simulink model "smartCart5_1work"  (R2016a)
settings: Solver=FixedStepDiscrete  StartTime=0.0  StopTime=inf  FixedStep=1  RelTol=1e-3
libraries: simulink x213, hdlsllib x84
(part 4 of 4)

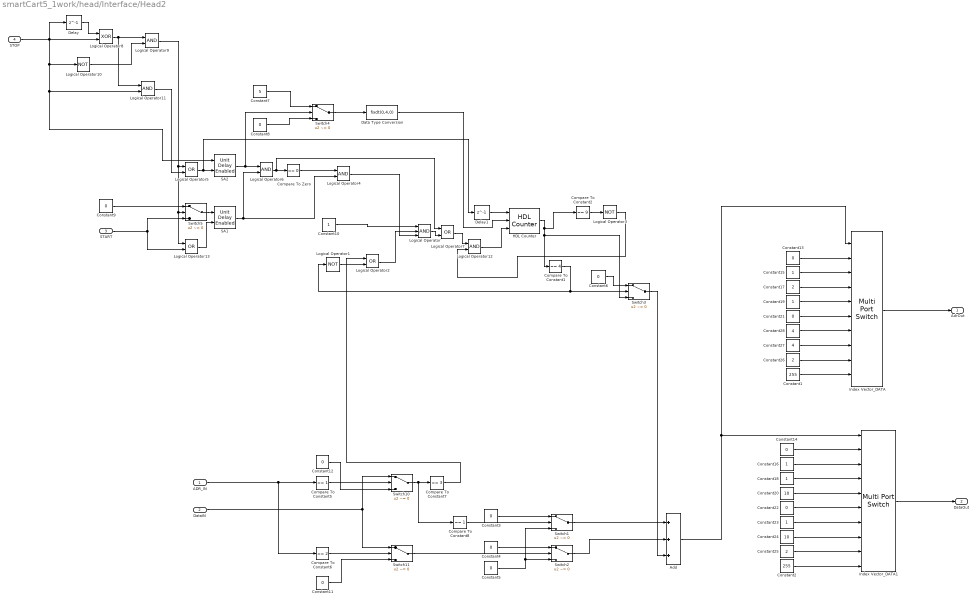
== system smartCart5_1work/head/Interface/Head2 ==
  ADR_IN : Inport  OutDataTypeStr=uint8
  DataIN : Inport  Port=2  OutDataTypeStr=uint8
  START : Inport  Port=3  OutDataTypeStr=boolean
  STOP : Inport  Port=4  OutDataTypeStr=boolean
  Add : Sum  Inputs=+++
  Compare To Constant1 : simulink/Logic and Bit Operations/Compare To Constant  relop===  const=4  OutDataTypeStr=boolean
  Compare To Constant2 : simulink/Logic and Bit Operations/Compare To Constant  relop===  const=9  OutDataTypeStr=boolean
  Compare To Constant5 : simulink/Logic and Bit Operations/Compare To Constant  relop===  const=1  OutDataTypeStr=boolean
  Compare To Constant6 : simulink/Logic and Bit Operations/Compare To Constant  relop===  const=2  OutDataTypeStr=boolean
  Compare To Constant7 : simulink/Logic and Bit Operations/Compare To Constant  relop===  const=3  OutDataTypeStr=boolean
  Compare To Constant8 : simulink/Logic and Bit Operations/Compare To Constant  relop===  const=1  OutDataTypeStr=boolean
  Compare To Zero : simulink/Logic and Bit Operations/Compare To Zero  relop===  OutDataTypeStr=boolean
  Constant1 : Constant  Value=255  OutDataTypeStr=uint8
  Constant10 : Constant  OutDataTypeStr=boolean
  Constant{3..6,11..14,21..22} (10 alike) : Constant  Value=0  OutDataTypeStr=uint8
  Constant{15..16,18..19,23} (5 alike) : Constant  OutDataTypeStr=uint8
  Constant17 : Constant  Value=2  OutDataTypeStr=uint8
  Constant2 : Constant  Value=255  OutDataTypeStr=uint8
  Constant20 : Constant  Value=10  OutDataTypeStr=uint8
  Constant24 : Constant  Value=10  OutDataTypeStr=uint8
  Constant25 : Constant  Value=2  OutDataTypeStr=uint8
  Constant26 : Constant  Value=2  OutDataTypeStr=uint8
  Constant27 : Constant  Value=4  OutDataTypeStr=uint8
  Constant28 : Constant  Value=4  OutDataTypeStr=uint8
  Constant7 : Constant  Value=5  OutDataTypeStr=fixdt(0,4,0)
  Constant8 : Constant  Value=0  OutDataTypeStr=fixdt(0,4,0)
  Constant9 : Constant  Value=0  OutDataTypeStr=boolean
  Data Type Conversion : DataTypeConversion  OutDataTypeStr=fixdt(0,4,0)
  Delay : Delay  DelayLength=1  InitialCondition=0
  Delay1 : Delay  DelayLength=1  InitialCondition=0
  HDL Counter : hdlsllib/HDL Operations/HDL Counter  CountType=Free running  CountInit=0  CountStep=1  CountMax=100  CountFromType=Initial value  CountFrom=0  CountResetPort=off  CountLoadPort=on  CountEnbPort=on  CountDirPort=off  CountDataType=Unsigned  CountWordLen=4  CountFracLen=0  CountSampTime=1
  Index Vector_DATA : MultiPortSwitch  DataPortOrder=Zero-based contiguous  Inputs=9  DiagnosticForDefault=None  zeroidx=on  OutDataTypeStr=uint8
  Index Vector_DATA1 : MultiPortSwitch  DataPortOrder=Zero-based contiguous  Inputs=9  DiagnosticForDefault=None  zeroidx=on  OutDataTypeStr=uint8
  Logical Operator : Logic  Inputs=3  AllPortsSameDT=off  OutDataTypeStr=boolean
  Logical Operator1 : Logic  Operator=NOT  AllPortsSameDT=off  OutDataTypeStr=boolean
  Logical Operator10 : Logic  Operator=NOT  AllPortsSameDT=off  OutDataTypeStr=boolean
  Logical Operator{4,6,9,11..12} (5 alike) : Logic  AllPortsSameDT=off  OutDataTypeStr=boolean
  Logical Operator{2,5,7,13} (4 alike) : Logic  Operator=OR  AllPortsSameDT=off  OutDataTypeStr=boolean
  Logical Operator3 : Logic  Operator=NOT  AllPortsSameDT=off  OutDataTypeStr=boolean
  Logical Operator8 : Logic  Operator=XOR  AllPortsSameDT=off  OutDataTypeStr=boolean
  SA1 : simulink/Additional Math & Discrete/Additional Discrete/Unit Delay Enabled  vinit=0  tsamp=-1
  SA2 : simulink/Additional Math & Discrete/Additional Discrete/Unit Delay Enabled  vinit=0  tsamp=-1
  Switch{1..5,10..11} (7 alike) : Switch  Criteria=u2 ~= 0  OutDataTypeStr=uint8
  AdrOut : Outport  OutDataTypeStr=uint8
  DataOut : Outport  Port=2  OutDataTypeStr=uint8
  wires:
  Constant10/1 -> Logical Operator/1
  Compare To Constant5/1 -> Switch10/2
  Compare To Constant6/1 -> Switch11/2
  Constant11/1 -> Switch11/3
  Constant12/1 -> Switch10/3
  Switch10/1 -> Compare To Constant8/1, Compare To Constant7/1
  Constant13/1 -> Index Vector_DATA/2
  Constant14/1 -> Index Vector_DATA1/2
  Constant15/1 -> Index Vector_DATA/3
  Constant16/1 -> Index Vector_DATA1/3
  Constant17/1 -> Index Vector_DATA/4
  Constant18/1 -> Index Vector_DATA1/4
  Constant19/1 -> Index Vector_DATA/5
  Constant20/1 -> Index Vector_DATA1/5
  Constant21/1 -> Index Vector_DATA/6
  Constant22/1 -> Index Vector_DATA1/6
  Constant23/1 -> Index Vector_DATA1/7
  Constant24/1 -> Index Vector_DATA1/8
  Constant25/1 -> Index Vector_DATA1/9
  Constant26/1 -> Index Vector_DATA/9
  Constant27/1 -> Index Vector_DATA/8
  Constant28/1 -> Index Vector_DATA/7
  Compare To Constant1/1 -> Logical Operator1/1, Switch3/2
  Compare To Constant7/1 -> Logical Operator2/1
  Logical Operator1/1 -> Logical Operator2/2
  Constant1/1 -> Index Vector_DATA/10
  Constant2/1 -> Index Vector_DATA1/10
  Logical Operator2/1 -> Logical Operator/2
  Compare To Constant8/1 -> Switch1/2
  Constant3/1 -> Switch1/1
  Switch11/1 -> Switch2/2
  Constant4/1 -> Switch2/1
  HDL Counter/1 -> Compare To Constant2/1, Switch3/3, Compare To Constant1/1
  Constant5/1 -> Switch1/3, Switch2/3
  Constant6/1 -> Switch3/1
  Switch1/1 -> Add/1
  Switch2/1 -> Add/2
  Switch3/1 -> Add/3
  Add/1 -> Index Vector_DATA/1, Index Vector_DATA1/1
  Index Vector_DATA1/1 -> DataOut/1
  Index Vector_DATA/1 -> AdrOut/1
  ADR_IN/1 -> Compare To Constant5/1, Compare To Constant6/1
  DataIN/1 -> Switch11/1, Switch10/1
  Compare To Constant2/1 -> Logical Operator3/1
  Compare To Zero/1 -> Logical Operator4/1
  SA1/1 -> Logical Operator6/2, Logical Operator4/2
  Logical Operator4/1 -> Logical Operator/3
  Logical Operator/1 -> Logical Operator7/2
  STOP/1 -> SA2/1, Logical Operator11/2, Logical Operator10/1, Delay/1, Logical Operator8/2
  Delay/1 -> Logical Operator8/1
  Logical Operator8/1 -> Logical Operator11/1, Logical Operator9/1
  Logical Operator10/1 -> Logical Operator9/2
  Logical Operator5/1 -> Delay1/1, SA2/2
  Logical Operator11/1 -> Logical Operator5/2
  Logical Operator9/1 -> Logical Operator13/1, Switch5/2, Logical Operator5/1
  SA2/1 -> Switch4/2, Logical Operator6/1
  Logical Operator6/1 -> Logical Operator7/1, Compare To Zero/1
  Constant7/1 -> Switch4/1
  Constant8/1 -> Switch4/3
  Switch4/1 -> Data Type Conversion/1
  Data Type Conversion/1 -> HDL Counter/2
  Delay1/1 -> HDL Counter/1
  Logical Operator12/1 -> HDL Counter/3
  Logical Operator3/1 -> Logical Operator12/2
  Logical Operator7/1 -> Logical Operator12/1
  Switch5/1 -> SA1/1
  Constant9/1 -> Switch5/1
  START/1 -> Logical Operator13/2, Switch5/3
  Logical Operator13/1 -> SA1/2

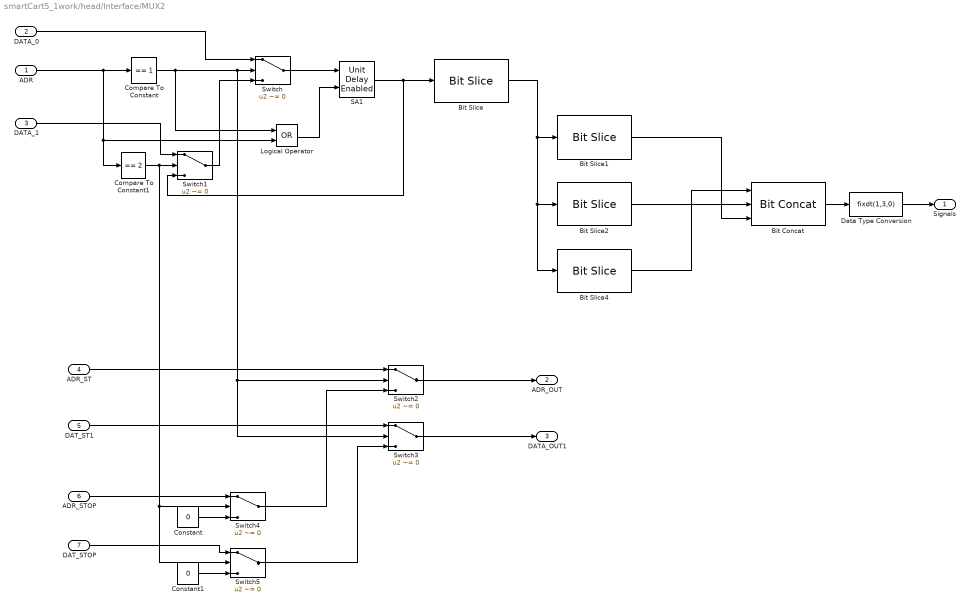
== system smartCart5_1work/head/Interface/MUX2 ==
  ADR : Inport  OutDataTypeStr=uint8
  DATA_0 : Inport  Port=2  OutDataTypeStr=uint8
  DATA_1 : Inport  Port=3  OutDataTypeStr=uint8
  ADR_ST : Inport  Port=4  OutDataTypeStr=uint8
  DAT_ST1 : Inport  Port=5  OutDataTypeStr=uint8
  ADR_STOP : Inport  Port=6  OutDataTypeStr=uint8
  DAT_STOP : Inport  Port=7  OutDataTypeStr=uint8
  Bit Concat : hdlsllib/HDL Operations/Bit Concat  numInputs=3
  Bit Slice : hdlsllib/HDL Operations/Bit Slice  lidx=4  ridx=0
  Bit Slice1 : hdlsllib/HDL Operations/Bit Slice  lidx=0  ridx=0
  Bit Slice2 : hdlsllib/HDL Operations/Bit Slice  lidx=1  ridx=1
  Bit Slice4 : hdlsllib/HDL Operations/Bit Slice  lidx=3  ridx=3
  Compare To Constant : simulink/Logic and Bit Operations/Compare To Constant  relop===  const=1  OutDataTypeStr=boolean
  Compare To Constant1 : simulink/Logic and Bit Operations/Compare To Constant  relop===  const=2  OutDataTypeStr=boolean
  Constant : Constant  Value=0  OutDataTypeStr=boolean
  Constant1 : Constant  Value=0  OutDataTypeStr=boolean
  Data Type Conversion : DataTypeConversion  OutDataTypeStr=fixdt(1,3,0)
  Logical Operator : Logic  Operator=OR  AllPortsSameDT=off  OutDataTypeStr=boolean
  SA1 : simulink/Additional Math & Discrete/Additional Discrete/Unit Delay Enabled  vinit=0  tsamp=-1
  Switch{,1..5} (6 alike) : Switch  Criteria=u2 ~= 0  OutDataTypeStr=uint8
  Signals : Outport  OutDataTypeStr=fixdt(1,3,0)
  ADR_OUT : Outport  Port=2  OutDataTypeStr=uint8
  DATA_OUT1 : Outport  Port=3  OutDataTypeStr=uint8
  wires:
  Bit Slice/1 -> Bit Slice4/1, Bit Slice2/1, Bit Slice1/1
  Compare To Constant/1 -> Logical Operator/1, Switch2/2, Switch3/2, Switch/2
  Switch1/1 -> Switch/3
  Compare To Constant1/1 -> Switch1/2, Switch4/2, Switch5/2
  Switch/1 -> SA1/1
  SA1/1 -> Bit Slice/1, Switch1/3
  Switch4/1 -> Switch2/3
  Switch5/1 -> Switch3/3
  Constant/1 -> Switch4/3
  Constant1/1 -> Switch5/3
  Logical Operator/1 -> SA1/2
  Switch2/1 -> ADR_OUT/1
  Switch3/1 -> DATA_OUT1/1
  DATA_0/1 -> Switch/1
  ADR/1 -> Logical Operator/2, Compare To Constant1/1, Compare To Constant/1
  DATA_1/1 -> Switch1/1
  ADR_ST/1 -> Switch2/1
  DAT_ST1/1 -> Switch3/1
  ADR_STOP/1 -> Switch4/1
  DAT_STOP/1 -> Switch5/1
  Bit Slice4/1 -> Bit Concat/1
  Bit Slice2/1 -> Bit Concat/2
  Bit Slice1/1 -> Bit Concat/3
  Bit Concat/1 -> Data Type Conversion/1
  Data Type Conversion/1 -> Signals/1

== system smartCart5_1work/head/Interface/Swith_signal2 ==
  Adr : Inport  OutDataTypeStr=uint8
  Data : Inport  Port=2  OutDataTypeStr=uint8
  Compare To Constant : simulink/Logic and Bit Operations/Compare To Constant  relop===  const=2  OutDataTypeStr=boolean
  SA1 : simulink/Additional Math & Discrete/Additional Discrete/Unit Delay Enabled  vinit=0  tsamp=-1
  OutAddr : Outport  OutDataTypeStr=uint8
  wires:
  Compare To Constant/1 -> SA1/2
  Adr/1 -> Compare To Constant/1
  Data/1 -> SA1/1
  SA1/1 -> OutAddr/1

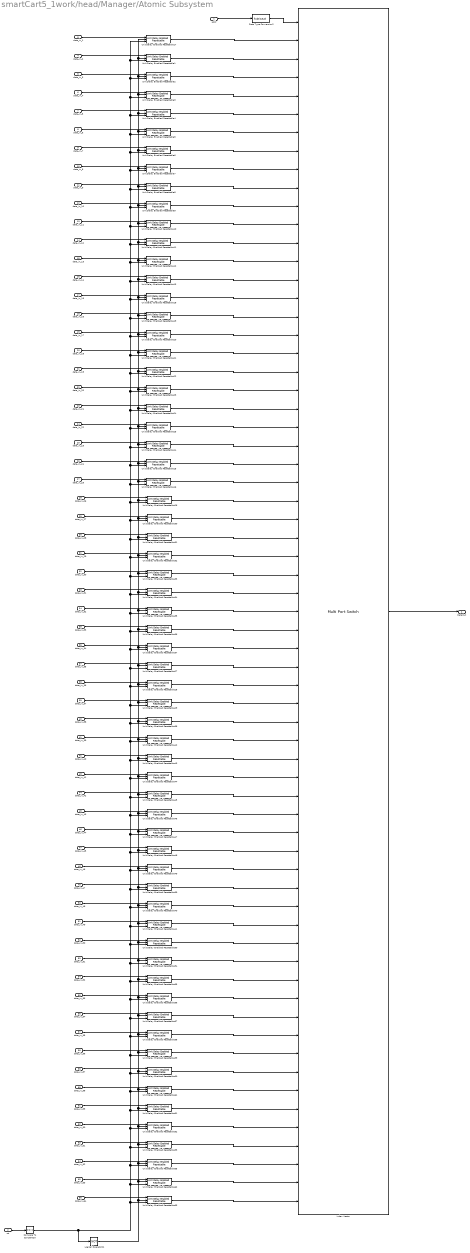
== system smartCart5_1work/head/Manager/Atomic Subsystem ==
  addr : Inport  OutDataTypeStr=uint8
  rst : Inport  Port=2  OutDataTypeStr=boolean
  data_in_1 : Inport  Port=3  OutDataTypeStr=uint32
  data_in_2 : Inport  Port=4  OutDataTypeStr=uint32
  data_in_3 : Inport  Port=5  OutDataTypeStr=uint32
  data_in_4 : Inport  Port=6  OutDataTypeStr=uint32
  data_in_5 : Inport  Port=7  OutDataTypeStr=uint32
  data_in_6 : Inport  Port=8  OutDataTypeStr=uint32
  data_in_7 : Inport  Port=9  OutDataTypeStr=uint32
  data_in_8 : Inport  Port=10  OutDataTypeStr=uint32
  data_in_9 : Inport  Port=11  OutDataTypeStr=uint32
  data_in_10 : Inport  Port=12  OutDataTypeStr=uint32
  data_in_11 : Inport  Port=13  OutDataTypeStr=uint32
  data_in_12 : Inport  Port=14  OutDataTypeStr=uint32
  data_in_13 : Inport  Port=15  OutDataTypeStr=uint32
  data_in_14 : Inport  Port=16  OutDataTypeStr=uint32
  data_in_15 : Inport  Port=17  OutDataTypeStr=uint32
  data_in_16 : Inport  Port=18  OutDataTypeStr=uint32
  data_in_17 : Inport  Port=19  OutDataTypeStr=uint32
  data_in_18 : Inport  Port=20  OutDataTypeStr=uint32
  data_in_19 : Inport  Port=21  OutDataTypeStr=uint32
  data_in_20 : Inport  Port=22  OutDataTypeStr=uint32
  data_in_21 : Inport  Port=23  OutDataTypeStr=uint32
  data_in_22 : Inport  Port=24  OutDataTypeStr=uint32
  data_in_23 : Inport  Port=25  OutDataTypeStr=uint32
  data_in_24 : Inport  Port=26  OutDataTypeStr=uint32
  data_in_25 : Inport  Port=27  OutDataTypeStr=uint32
  data_in_26 : Inport  Port=28  OutDataTypeStr=uint32
  data_in_27 : Inport  Port=29  OutDataTypeStr=uint32
  data_in_28 : Inport  Port=30  OutDataTypeStr=uint32
  data_in_29 : Inport  Port=31  OutDataTypeStr=uint32
  data_in_30 : Inport  Port=32  OutDataTypeStr=uint32
  data_in_31 : Inport  Port=33  OutDataTypeStr=uint32
  data_in_32 : Inport  Port=34  OutDataTypeStr=uint32
  data_in_33 : Inport  Port=35  OutDataTypeStr=uint32
  data_in_34 : Inport  Port=36  OutDataTypeStr=uint32
  data_in_35 : Inport  Port=37  OutDataTypeStr=uint32
  data_in_36 : Inport  Port=38  OutDataTypeStr=uint32
  data_in_37 : Inport  Port=39  OutDataTypeStr=uint32
  data_in_38 : Inport  Port=40  OutDataTypeStr=uint32
  data_in_39 : Inport  Port=41  OutDataTypeStr=uint32
  data_in_40 : Inport  Port=42  OutDataTypeStr=uint32
  data_in_41 : Inport  Port=43  OutDataTypeStr=uint32
  data_in_42 : Inport  Port=44  OutDataTypeStr=uint32
  data_in_43 : Inport  Port=45  OutDataTypeStr=uint32
  data_in_44 : Inport  Port=46  OutDataTypeStr=uint32
  data_in_45 : Inport  Port=47  OutDataTypeStr=uint32
  data_in_46 : Inport  Port=48  OutDataTypeStr=uint32
  data_in_47 : Inport  Port=49  OutDataTypeStr=uint32
  data_in_48 : Inport  Port=50  OutDataTypeStr=uint32
  data_in_49 : Inport  Port=51  OutDataTypeStr=uint32
  data_in_50 : Inport  Port=52  OutDataTypeStr=uint32
  data_in_51 : Inport  Port=53  OutDataTypeStr=uint32
  data_in_52 : Inport  Port=54  OutDataTypeStr=uint32
  data_in_53 : Inport  Port=55  OutDataTypeStr=uint32
  data_in_54 : Inport  Port=56  OutDataTypeStr=uint32
  data_in_55 : Inport  Port=57  OutDataTypeStr=uint32
  data_in_56 : Inport  Port=58  OutDataTypeStr=uint32
  data_in_57 : Inport  Port=59  OutDataTypeStr=uint32
  data_in_58 : Inport  Port=60  OutDataTypeStr=uint32
  data_in_59 : Inport  Port=61  OutDataTypeStr=uint32
  data_in_60 : Inport  Port=62  OutDataTypeStr=uint32
  data_in_61 : Inport  Port=63  OutDataTypeStr=uint32
  data_in_62 : Inport  Port=64  OutDataTypeStr=uint32
  data_in_63 : Inport  Port=65  OutDataTypeStr=uint32
  data_in_64 : Inport  Port=66  OutDataTypeStr=uint32
  Compare To Constant20 : simulink/Logic and Bit Operations/Compare To Constant  relop===  const=1  OutDataTypeStr=boolean
  Data Type Conversion2 : DataTypeConversion  OutDataTypeStr=fixdt(0,6,0)
  Index Vector : MultiPortSwitch  DataPortOrder=Zero-based contiguous  Inputs=64  zeroidx=on
  Logical Operator21 : Logic  Operator=NOT  AllPortsSameDT=off  OutDataTypeStr=boolean
  Unit Delay Enabled Resettable{1..63,65} (64 alike) : simulink/Additional Math & Discrete/Additional Discrete/Unit Delay Enabled Resettable  vinit=0  tsamp=-1
  DataOut : Outport  OutDataTypeStr=uint32
  wires:
  addr/1 -> Data Type Conversion2/1
  data_in_1/1 -> Unit Delay Enabled Resettable17/1
  Unit Delay Enabled Resettable17/1 -> Index Vector/2
  rst/1 -> Compare To Constant20/1
  Unit Delay Enabled Resettable1/1 -> Index Vector/3
  Unit Delay Enabled Resettable2/1 -> Index Vector/4
  Unit Delay Enabled Resettable3/1 -> Index Vector/5
  Unit Delay Enabled Resettable4/1 -> Index Vector/6
  Unit Delay Enabled Resettable5/1 -> Index Vector/7
  Unit Delay Enabled Resettable6/1 -> Index Vector/8
  Unit Delay Enabled Resettable7/1 -> Index Vector/9
  Unit Delay Enabled Resettable8/1 -> Index Vector/10
  Unit Delay Enabled Resettable9/1 -> Index Vector/11
  Unit Delay Enabled Resettable10/1 -> Index Vector/12
  Unit Delay Enabled Resettable11/1 -> Index Vector/13
  Unit Delay Enabled Resettable12/1 -> Index Vector/14
  Unit Delay Enabled Resettable13/1 -> Index Vector/15
  Unit Delay Enabled Resettable18/1 -> Index Vector/16
  Unit Delay Enabled Resettable19/1 -> Index Vector/17
  Unit Delay Enabled Resettable20/1 -> Index Vector/18
  Unit Delay Enabled Resettable21/1 -> Index Vector/19
  Unit Delay Enabled Resettable22/1 -> Index Vector/20
  Unit Delay Enabled Resettable23/1 -> Index Vector/21
  Unit Delay Enabled Resettable24/1 -> Index Vector/22
  Unit Delay Enabled Resettable25/1 -> Index Vector/23
  Unit Delay Enabled Resettable14/1 -> Index Vector/24
  Unit Delay Enabled Resettable15/1 -> Index Vector/25
  Unit Delay Enabled Resettable16/1 -> Index Vector/26
  Unit Delay Enabled Resettable26/1 -> Index Vector/27
  Unit Delay Enabled Resettable30/1 -> Index Vector/28
  Unit Delay Enabled Resettable31/1 -> Index Vector/29
  Unit Delay Enabled Resettable32/1 -> Index Vector/30
  Unit Delay Enabled Resettable33/1 -> Index Vector/31
  Unit Delay Enabled Resettable34/1 -> Index Vector/32
  Unit Delay Enabled Resettable35/1 -> Index Vector/33
  Unit Delay Enabled Resettable36/1 -> Index Vector/34
  Unit Delay Enabled Resettable37/1 -> Index Vector/35
  Unit Delay Enabled Resettable27/1 -> Index Vector/36
  Unit Delay Enabled Resettable28/1 -> Index Vector/37
  Unit Delay Enabled Resettable29/1 -> Index Vector/38
  Unit Delay Enabled Resettable38/1 -> Index Vector/39
  Unit Delay Enabled Resettable42/1 -> Index Vector/40
  Unit Delay Enabled Resettable43/1 -> Index Vector/41
  Unit Delay Enabled Resettable44/1 -> Index Vector/42
  Unit Delay Enabled Resettable45/1 -> Index Vector/43
  Unit Delay Enabled Resettable46/1 -> Index Vector/44
  Unit Delay Enabled Resettable47/1 -> Index Vector/45
  Unit Delay Enabled Resettable48/1 -> Index Vector/46
  Unit Delay Enabled Resettable49/1 -> Index Vector/47
  Unit Delay Enabled Resettable39/1 -> Index Vector/48
  Unit Delay Enabled Resettable40/1 -> Index Vector/49
  Unit Delay Enabled Resettable41/1 -> Index Vector/50
  Unit Delay Enabled Resettable50/1 -> Index Vector/51
  Unit Delay Enabled Resettable54/1 -> Index Vector/52
  Unit Delay Enabled Resettable55/1 -> Index Vector/53
  Unit Delay Enabled Resettable56/1 -> Index Vector/54
  Unit Delay Enabled Resettable57/1 -> Index Vector/55
  Unit Delay Enabled Resettable58/1 -> Index Vector/56
  Unit Delay Enabled Resettable59/1 -> Index Vector/57
  Unit Delay Enabled Resettable60/1 -> Index Vector/58
  Unit Delay Enabled Resettable61/1 -> Index Vector/59
  Unit Delay Enabled Resettable51/1 -> Index Vector/60
  Unit Delay Enabled Resettable52/1 -> Index Vector/61
  Unit Delay Enabled Resettable53/1 -> Index Vector/62
  Unit Delay Enabled Resettable65/1 -> Index Vector/63
  Unit Delay Enabled Resettable62/1 -> Index Vector/64
  Unit Delay Enabled Resettable63/1 -> Index Vector/65
  Data Type Conversion2/1 -> Index Vector/1
  data_in_2/1 -> Unit Delay Enabled Resettable1/1
  data_in_3/1 -> Unit Delay Enabled Resettable2/1
  data_in_4/1 -> Unit Delay Enabled Resettable3/1
  data_in_5/1 -> Unit Delay Enabled Resettable4/1
  data_in_6/1 -> Unit Delay Enabled Resettable5/1
  data_in_7/1 -> Unit Delay Enabled Resettable6/1
  data_in_8/1 -> Unit Delay Enabled Resettable7/1
  data_in_9/1 -> Unit Delay Enabled Resettable8/1
  data_in_10/1 -> Unit Delay Enabled Resettable9/1
  data_in_11/1 -> Unit Delay Enabled Resettable10/1
  data_in_12/1 -> Unit Delay Enabled Resettable11/1
  data_in_13/1 -> Unit Delay Enabled Resettable12/1
  data_in_14/1 -> Unit Delay Enabled Resettable13/1
  data_in_15/1 -> Unit Delay Enabled Resettable18/1
  data_in_16/1 -> Unit Delay Enabled Resettable19/1
  data_in_17/1 -> Unit Delay Enabled Resettable20/1
  data_in_18/1 -> Unit Delay Enabled Resettable21/1
  data_in_19/1 -> Unit Delay Enabled Resettable22/1
  data_in_20/1 -> Unit Delay Enabled Resettable23/1
  data_in_21/1 -> Unit Delay Enabled Resettable24/1
  data_in_22/1 -> Unit Delay Enabled Resettable25/1
  data_in_23/1 -> Unit Delay Enabled Resettable14/1
  data_in_24/1 -> Unit Delay Enabled Resettable15/1
  data_in_25/1 -> Unit Delay Enabled Resettable16/1
  data_in_26/1 -> Unit Delay Enabled Resettable26/1
  data_in_27/1 -> Unit Delay Enabled Resettable30/1
  data_in_28/1 -> Unit Delay Enabled Resettable31/1
  data_in_29/1 -> Unit Delay Enabled Resettable32/1
  data_in_30/1 -> Unit Delay Enabled Resettable33/1
  data_in_31/1 -> Unit Delay Enabled Resettable34/1
  data_in_32/1 -> Unit Delay Enabled Resettable35/1
  data_in_33/1 -> Unit Delay Enabled Resettable36/1
  data_in_34/1 -> Unit Delay Enabled Resettable37/1
  data_in_35/1 -> Unit Delay Enabled Resettable27/1
  data_in_36/1 -> Unit Delay Enabled Resettable28/1
  data_in_37/1 -> Unit Delay Enabled Resettable29/1
  data_in_38/1 -> Unit Delay Enabled Resettable38/1
  data_in_39/1 -> Unit Delay Enabled Resettable42/1
  data_in_40/1 -> Unit Delay Enabled Resettable43/1
  data_in_41/1 -> Unit Delay Enabled Resettable44/1
  data_in_42/1 -> Unit Delay Enabled Resettable45/1
  data_in_43/1 -> Unit Delay Enabled Resettable46/1
  data_in_44/1 -> Unit Delay Enabled Resettable47/1
  data_in_45/1 -> Unit Delay Enabled Resettable48/1
  data_in_46/1 -> Unit Delay Enabled Resettable49/1
  data_in_47/1 -> Unit Delay Enabled Resettable39/1
  data_in_48/1 -> Unit Delay Enabled Resettable40/1
  data_in_49/1 -> Unit Delay Enabled Resettable41/1
  data_in_50/1 -> Unit Delay Enabled Resettable50/1
  data_in_51/1 -> Unit Delay Enabled Resettable54/1
  data_in_52/1 -> Unit Delay Enabled Resettable55/1
  data_in_53/1 -> Unit Delay Enabled Resettable56/1
  data_in_54/1 -> Unit Delay Enabled Resettable57/1
  data_in_55/1 -> Unit Delay Enabled Resettable58/1
  data_in_56/1 -> Unit Delay Enabled Resettable59/1
  data_in_57/1 -> Unit Delay Enabled Resettable60/1
  data_in_58/1 -> Unit Delay Enabled Resettable61/1
  data_in_59/1 -> Unit Delay Enabled Resettable51/1
  data_in_60/1 -> Unit Delay Enabled Resettable52/1
  data_in_61/1 -> Unit Delay Enabled Resettable53/1
  data_in_62/1 -> Unit Delay Enabled Resettable65/1
  data_in_63/1 -> Unit Delay Enabled Resettable62/1
  data_in_64/1 -> Unit Delay Enabled Resettable63/1
  Compare To Constant20/1 -> Logical Operator21/1, Unit Delay Enabled Resettable63/3, Unit Delay Enabled Resettable62/3, Unit Delay Enabled Resettable65/3, Unit Delay Enabled Resettable53/3, Unit Delay Enabled Resettable52/3, Unit Delay Enabled Resettable51/3, Unit Delay Enabled Resettable61/3, Unit Delay Enabled Resettable60/3, Unit Delay Enabled Resettable59/3, Unit Delay Enabled Resettable58/3, Unit Delay Enabled Resettable57/3, Unit Delay Enabled Resettable56/3, Unit Delay Enabled Resettable55/3, Unit Delay Enabled Resettable54/3, Unit Delay Enabled Resettable50/3, Unit Delay Enabled Resettable41/3, Unit Delay Enabled Resettable40/3, Unit Delay Enabled Resettable39/3, Unit Delay Enabled Resettable49/3, Unit Delay Enabled Resettable48/3, Unit Delay Enabled Resettable47/3, Unit Delay Enabled Resettable46/3, Unit Delay Enabled Resettable45/3, Unit Delay Enabled Resettable44/3, Unit Delay Enabled Resettable43/3, Unit Delay Enabled Resettable42/3, Unit Delay Enabled Resettable38/3, Unit Delay Enabled Resettable29/3, Unit Delay Enabled Resettable28/3, Unit Delay Enabled Resettable27/3, Unit Delay Enabled Resettable37/3, Unit Delay Enabled Resettable36/3, Unit Delay Enabled Resettable35/3, Unit Delay Enabled Resettable34/3, Unit Delay Enabled Resettable33/3, Unit Delay Enabled Resettable32/3, Unit Delay Enabled Resettable31/3, Unit Delay Enabled Resettable30/3, Unit Delay Enabled Resettable26/3, Unit Delay Enabled Resettable16/3, Unit Delay Enabled Resettable15/3, Unit Delay Enabled Resettable14/3, Unit Delay Enabled Resettable25/3, Unit Delay Enabled Resettable24/3, Unit Delay Enabled Resettable23/3, Unit Delay Enabled Resettable22/3, Unit Delay Enabled Resettable21/3, Unit Delay Enabled Resettable20/3, Unit Delay Enabled Resettable19/3, Unit Delay Enabled Resettable18/3, Unit Delay Enabled Resettable13/3, Unit Delay Enabled Resettable12/3, Unit Delay Enabled Resettable11/3, Unit Delay Enabled Resettable10/3, Unit Delay Enabled Resettable9/3, Unit Delay Enabled Resettable8/3, Unit Delay Enabled Resettable7/3, Unit Delay Enabled Resettable6/3, Unit Delay Enabled Resettable5/3, Unit Delay Enabled Resettable4/3, Unit Delay Enabled Resettable3/3, Unit Delay Enabled Resettable2/3, Unit Delay Enabled Resettable1/3, Unit Delay Enabled Resettable17/3
  Logical Operator21/1 -> Unit Delay Enabled Resettable51/2, Unit Delay Enabled Resettable58/2, Unit Delay Enabled Resettable55/2, Unit Delay Enabled Resettable41/2, Unit Delay Enabled Resettable39/2, Unit Delay Enabled Resettable49/2, Unit Delay Enabled Resettable48/2, Unit Delay Enabled Resettable46/2, Unit Delay Enabled Resettable44/2, Unit Delay Enabled Resettable43/2, Unit Delay Enabled Resettable29/2, Unit Delay Enabled Resettable28/2, Unit Delay Enabled Resettable27/2, Unit Delay Enabled Resettable37/2, Unit Delay Enabled Resettable36/2, Unit Delay Enabled Resettable35/2, Unit Delay Enabled Resettable32/2, Unit Delay Enabled Resettable16/2, Unit Delay Enabled Resettable15/2, Unit Delay Enabled Resettable14/2, Unit Delay Enabled Resettable25/2, Unit Delay Enabled Resettable21/2, Unit Delay Enabled Resettable13/2, Unit Delay Enabled Resettable12/2, Unit Delay Enabled Resettable11/2, Unit Delay Enabled Resettable10/2, Unit Delay Enabled Resettable9/2, Unit Delay Enabled Resettable8/2, Unit Delay Enabled Resettable7/2, Unit Delay Enabled Resettable6/2, Unit Delay Enabled Resettable5/2, Unit Delay Enabled Resettable4/2, Unit Delay Enabled Resettable3/2, Unit Delay Enabled Resettable2/2, Unit Delay Enabled Resettable1/2, Unit Delay Enabled Resettable17/2, Unit Delay Enabled Resettable18/2, Unit Delay Enabled Resettable19/2, Unit Delay Enabled Resettable20/2, Unit Delay Enabled Resettable22/2, Unit Delay Enabled Resettable23/2, Unit Delay Enabled Resettable24/2, Unit Delay Enabled Resettable26/2, Unit Delay Enabled Resettable30/2, Unit Delay Enabled Resettable31/2, Unit Delay Enabled Resettable33/2, Unit Delay Enabled Resettable34/2, Unit Delay Enabled Resettable38/2, Unit Delay Enabled Resettable42/2, Unit Delay Enabled Resettable45/2, Unit Delay Enabled Resettable47/2, Unit Delay Enabled Resettable40/2, Unit Delay Enabled Resettable50/2, Unit Delay Enabled Resettable54/2, Unit Delay Enabled Resettable56/2, Unit Delay Enabled Resettable57/2, Unit Delay Enabled Resettable59/2, Unit Delay Enabled Resettable60/2, Unit Delay Enabled Resettable61/2, Unit Delay Enabled Resettable52/2, Unit Delay Enabled Resettable53/2, Unit Delay Enabled Resettable65/2, Unit Delay Enabled Resettable62/2, Unit Delay Enabled Resettable63/2
  Index Vector/1 -> DataOut/1

== system smartCart5_1work/head/Manager/signal_edg ==
  In1 : Inport  OutDataTypeStr=boolean
  Delay4 : Delay  DelayLength=1  InitialCondition=0
  Logical Operator1 : Logic  Operator=XOR  AllPortsSameDT=off  OutDataTypeStr=boolean
  Logical Operator15 : Logic  AllPortsSameDT=off  OutDataTypeStr=boolean
  Out1 : Outport  OutDataTypeStr=boolean
  wires:
  Logical Operator15/1 -> Out1/1
  In1/1 -> Logical Operator1/2, Logical Operator15/2, Delay4/1
  Logical Operator1/1 -> Logical Operator15/1
  Delay4/1 -> Logical Operator1/1

== system smartCart5_1work/head/Manager/signal_edg1 ==
  In1 : Inport  OutDataTypeStr=boolean
  Delay4 : Delay  DelayLength=1  InitialCondition=0
  Logical Operator1 : Logic  Operator=XOR  AllPortsSameDT=off  OutDataTypeStr=boolean
  Logical Operator15 : Logic  AllPortsSameDT=off  OutDataTypeStr=boolean
  Out1 : Outport  OutDataTypeStr=boolean
  wires:
  Delay4/1 -> Logical Operator1/1
  Logical Operator1/1 -> Logical Operator15/1
  In1/1 -> Delay4/1, Logical Operator15/2, Logical Operator1/2
  Logical Operator15/1 -> Out1/1

== system smartCart5_1work/head/Manager/signal_edg10 ==
  In1 : Inport  OutDataTypeStr=boolean
  Delay4 : Delay  DelayLength=1  InitialCondition=0
  Logical Operator1 : Logic  Operator=XOR  AllPortsSameDT=off  OutDataTypeStr=boolean
  Logical Operator15 : Logic  AllPortsSameDT=off  OutDataTypeStr=boolean
  Out1 : Outport  OutDataTypeStr=boolean
  wires:
  Logical Operator15/1 -> Out1/1
  In1/1 -> Logical Operator1/2, Logical Operator15/2, Delay4/1
  Logical Operator1/1 -> Logical Operator15/1
  Delay4/1 -> Logical Operator1/1

== system smartCart5_1work/head/Manager/signal_edg11 ==
  In1 : Inport  OutDataTypeStr=boolean
  Delay4 : Delay  DelayLength=1  InitialCondition=0
  Logical Operator1 : Logic  Operator=XOR  AllPortsSameDT=off  OutDataTypeStr=boolean
  Logical Operator15 : Logic  AllPortsSameDT=off  OutDataTypeStr=boolean
  Out1 : Outport  OutDataTypeStr=boolean
  wires:
  Delay4/1 -> Logical Operator1/1
  Logical Operator1/1 -> Logical Operator15/1
  In1/1 -> Delay4/1, Logical Operator15/2, Logical Operator1/2
  Logical Operator15/1 -> Out1/1

== system smartCart5_1work/head/Manager/signal_edg12 ==
  In1 : Inport  OutDataTypeStr=boolean
  Delay4 : Delay  DelayLength=1  InitialCondition=0
  Logical Operator1 : Logic  Operator=XOR  AllPortsSameDT=off  OutDataTypeStr=boolean
  Logical Operator15 : Logic  AllPortsSameDT=off  OutDataTypeStr=boolean
  Out1 : Outport  OutDataTypeStr=boolean
  wires:
  Logical Operator15/1 -> Out1/1
  In1/1 -> Logical Operator1/2, Logical Operator15/2, Delay4/1
  Logical Operator1/1 -> Logical Operator15/1
  Delay4/1 -> Logical Operator1/1

== system smartCart5_1work/head/Manager/signal_edg2 ==
  In1 : Inport  OutDataTypeStr=boolean
  Delay4 : Delay  DelayLength=1  InitialCondition=0
  Logical Operator1 : Logic  Operator=XOR  AllPortsSameDT=off  OutDataTypeStr=boolean
  Logical Operator15 : Logic  AllPortsSameDT=off  OutDataTypeStr=boolean
  Out1 : Outport  OutDataTypeStr=boolean
  wires:
  Delay4/1 -> Logical Operator1/1
  Logical Operator1/1 -> Logical Operator15/1
  In1/1 -> Delay4/1, Logical Operator15/2, Logical Operator1/2
  Logical Operator15/1 -> Out1/1

== system smartCart5_1work/head/Manager/signal_edg3 ==
  In1 : Inport  OutDataTypeStr=boolean
  Delay4 : Delay  DelayLength=1  InitialCondition=0
  Logical Operator1 : Logic  Operator=XOR  AllPortsSameDT=off  OutDataTypeStr=boolean
  Logical Operator15 : Logic  AllPortsSameDT=off  OutDataTypeStr=boolean
  Out1 : Outport  OutDataTypeStr=boolean
  wires:
  Logical Operator15/1 -> Out1/1
  In1/1 -> Logical Operator1/2, Logical Operator15/2, Delay4/1
  Logical Operator1/1 -> Logical Operator15/1
  Delay4/1 -> Logical Operator1/1

== system smartCart5_1work/head/Manager/signal_edg4 ==
  In1 : Inport  OutDataTypeStr=boolean
  Delay4 : Delay  DelayLength=1  InitialCondition=0
  Logical Operator1 : Logic  Operator=XOR  AllPortsSameDT=off  OutDataTypeStr=boolean
  Logical Operator15 : Logic  AllPortsSameDT=off  OutDataTypeStr=boolean
  Out1 : Outport  OutDataTypeStr=boolean
  wires:
  Logical Operator15/1 -> Out1/1
  In1/1 -> Logical Operator1/2, Logical Operator15/2, Delay4/1
  Logical Operator1/1 -> Logical Operator15/1
  Delay4/1 -> Logical Operator1/1

== system smartCart5_1work/head/Manager/signal_edg6 ==
  In1 : Inport  OutDataTypeStr=boolean
  Delay4 : Delay  DelayLength=1  InitialCondition=0
  Logical Operator1 : Logic  Operator=XOR  AllPortsSameDT=off  OutDataTypeStr=boolean
  Logical Operator15 : Logic  AllPortsSameDT=off  OutDataTypeStr=boolean
  Out1 : Outport  OutDataTypeStr=boolean
  wires:
  Logical Operator15/1 -> Out1/1
  In1/1 -> Logical Operator1/2, Logical Operator15/2, Delay4/1
  Logical Operator1/1 -> Logical Operator15/1
  Delay4/1 -> Logical Operator1/1

== system smartCart5_1work/head/Manager/signal_edg7 ==
  In1 : Inport  OutDataTypeStr=boolean
  Delay4 : Delay  DelayLength=1  InitialCondition=0
  Logical Operator1 : Logic  Operator=XOR  AllPortsSameDT=off  OutDataTypeStr=boolean
  Logical Operator15 : Logic  AllPortsSameDT=off  OutDataTypeStr=boolean
  Out1 : Outport  OutDataTypeStr=boolean
  wires:
  Logical Operator15/1 -> Out1/1
  In1/1 -> Logical Operator1/2, Logical Operator15/2, Delay4/1
  Logical Operator1/1 -> Logical Operator15/1
  Delay4/1 -> Logical Operator1/1

== system smartCart5_1work/head/Manager/signal_edg8 ==
  In1 : Inport  OutDataTypeStr=boolean
  Delay4 : Delay  DelayLength=1  InitialCondition=0
  Logical Operator1 : Logic  Operator=XOR  AllPortsSameDT=off  OutDataTypeStr=boolean
  Logical Operator15 : Logic  AllPortsSameDT=off  OutDataTypeStr=boolean
  Out1 : Outport  OutDataTypeStr=boolean
  wires:
  Delay4/1 -> Logical Operator1/1
  Logical Operator1/1 -> Logical Operator15/1
  In1/1 -> Delay4/1, Logical Operator15/2, Logical Operator1/2
  Logical Operator15/1 -> Out1/1

== system smartCart5_1work/head/Manager/signal_edg9 ==
  In1 : Inport  OutDataTypeStr=boolean
  Delay4 : Delay  DelayLength=1  InitialCondition=0
  Logical Operator1 : Logic  Operator=XOR  AllPortsSameDT=off  OutDataTypeStr=boolean
  Logical Operator15 : Logic  AllPortsSameDT=off  OutDataTypeStr=boolean
  Out1 : Outport  OutDataTypeStr=boolean
  wires:
  Delay4/1 -> Logical Operator1/1
  Logical Operator1/1 -> Logical Operator15/1
  In1/1 -> Delay4/1, Logical Operator15/2, Logical Operator1/2
  Logical Operator15/1 -> Out1/1

== system smartCart5_1work/head/Reciver/signal_edg ==
  In1 : Inport  OutDataTypeStr=boolean
  Delay4 : Delay  DelayLength=1  InitialCondition=0
  Logical Operator1 : Logic  Operator=XOR  AllPortsSameDT=off  OutDataTypeStr=boolean
  Logical Operator15 : Logic  AllPortsSameDT=off  OutDataTypeStr=boolean
  Out1 : Outport  OutDataTypeStr=boolean
  wires:
  Logical Operator15/1 -> Out1/1
  In1/1 -> Logical Operator1/2, Logical Operator15/2, Delay4/1
  Logical Operator1/1 -> Logical Operator15/1
  Delay4/1 -> Logical Operator1/1

== system smartCart5_1work/head/Reciver/signal_edg5 ==
  In1 : Inport  OutDataTypeStr=boolean
  Delay4 : Delay  DelayLength=1  InitialCondition=0
  Logical Operator1 : Logic  Operator=XOR  AllPortsSameDT=off  OutDataTypeStr=boolean
  Logical Operator15 : Logic  AllPortsSameDT=off  OutDataTypeStr=boolean
  Out1 : Outport  OutDataTypeStr=boolean
  wires:
  Logical Operator15/1 -> Out1/1
  In1/1 -> Logical Operator1/2, Logical Operator15/2, Delay4/1
  Logical Operator1/1 -> Logical Operator15/1
  Delay4/1 -> Logical Operator1/1

== system smartCart5_1work/head/Reciver/signal_edg6 ==
  In1 : Inport  OutDataTypeStr=boolean
  Delay4 : Delay  DelayLength=1  InitialCondition=0
  Logical Operator1 : Logic  Operator=XOR  AllPortsSameDT=off  OutDataTypeStr=boolean
  Logical Operator15 : Logic  AllPortsSameDT=off  OutDataTypeStr=boolean
  Out1 : Outport  OutDataTypeStr=boolean
  wires:
  Logical Operator15/1 -> Out1/1
  In1/1 -> Logical Operator1/2, Logical Operator15/2, Delay4/1
  Logical Operator1/1 -> Logical Operator15/1
  Delay4/1 -> Logical Operator1/1
